simulink model "RCcircuit"  (R2019a)
settings: Solver=ode23t  StartTime=0.0  StopTime=2  MaxStep=1e-6  RelTol=1e-10
libraries: powerlib x7
settings Model: Creator=w0x7ce  LastModifiedBy=w0x7ce
settings SolverCC: AlgebraicLoopSolver=LineSearch

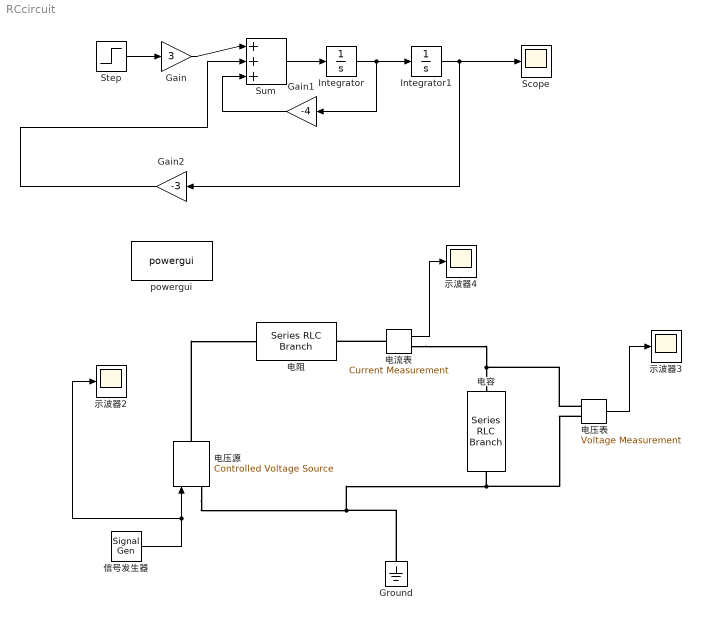
== system RCcircuit ==
  Gain : Gain  Gain=3
  Gain1 : Gain  Gain=-4
  Gain2 : Gain  Gain=-3
  Ground : powerlib/Elements/Ground  LConnTagsString=a
      settings: SourceProductName=Simscape Electrical
  Integrator : Integrator
  Integrator1 : Integrator
  Scope : Scope
  Step : Step  SampleTime=0
  Sum : Sum  Inputs=|+++
  powergui : powerlib/powergui  Priority=1  SimulationMode=Continuous  SampleTime=50e-6  frequency=60  Iterations=50  frequencyindice=0  Pbase=100e6  ErrMax=1e-4  UnitsV=kV  UnitsW=MW  buscounter=0  FunctionMessages=off  echomessages=off  EnableUseOfTLC=off  CurrentSourceSwitches=off  DisableSnubberDevices=off  DisableRonSwitches=off  DisableVfSwitches=off  DisplayEquations=off  AutomaticDiscreteSolvers=off  SolverType=Tustin/Backward Euler (TBE)  Interpol=off  ExternalGateDelay=off  methode=off  Ts=100  x0status=blocks  SPID=on  SwTol=0  HookPort=off  NonlinearTolerance=0  nMaxIteration=15  ContinueOnMaxIteration=off  RestoreLinks=warning  ResistiveCurrentMeasurement=off  Frange=[0:2:500]  Ylog=off  Xlog=on  ShowGrid=off  save=off  variable=ZData  structure=0  ZoomFFT=off  StartTime=0.0  cycles=1  DisplayStyle=1  fundamental=60  FreqAxis=off  MaxFrequency=1000  frequencyindicesteady=1  RmsSteady=1  display=off
      settings: SourceProductName=Simscape Electrical
  信号发生器 : SignalGenerator  WaveForm=square  Amplitude=10  Frequency=2
  电压源 : powerlib/Electrical Sources/Controlled Voltage Source  Initialize=on  Source_Type=AC  Amplitude=0  Phase=0  Frequency=0  Measurements=None
      settings: SourceProductName=Simscape Electrical
  电压表 : powerlib/Measurements/Voltage Measurement  PhasorSimulation=off  OutputType=Complex  PSBequivalent=0
      settings: SourceProductName=Simscape Electrical
  电容 : powerlib/Elements/Series RLC Branch  LConnTagsString=__new0  RConnTagsString=__new0  BranchType=C  Resistance=1  Inductance=1e-3  SetiL0=off  InitialCurrent=0  Capacitance=1e-6  Setx0=off  InitialVoltage=0  Measurements=None
      settings: SourceProductName=Simscape Electrical
  电流表 : powerlib/Measurements/Current Measurement  PhasorSimulation=off  OutputType=Complex  PSBequivalent=0
      settings: SourceProductName=Simscape Electrical
  电阻 : powerlib/Elements/Series RLC Branch  LConnTagsString=__new0  RConnTagsString=__new0  BranchType=R  Resistance=1  Inductance=1e-3  SetiL0=off  InitialCurrent=0  Capacitance=1e-6  Setx0=off  InitialVoltage=0  Measurements=None
      settings: SourceProductName=Simscape Electrical
  示波器2 : Scope
  示波器3 : Scope
  示波器4 : Scope
  wires:
  Step/1 -> Gain/1
  Gain/1 -> Sum/1
  Gain1/1 -> Sum/3
  Gain2/1 -> Sum/2
  Integrator/1 -> Gain1/1, Integrator1/1
  Sum/1 -> Integrator/1
  Integrator1/1 -> Scope/1, Gain2/1
  信号发生器/1 -> 示波器2/1, 电压源/1
  电压表/1 -> 示波器3/1
  电流表/1 -> 示波器4/1
  connections:
  电压源/RConn1 -- 电阻/LConn1
  电压源/LConn1 -- Ground/LConn1 -- 电压表/LConn2 -- 电容/RConn1
  电流表/LConn1 -- 电阻/RConn1
  电流表/RConn1 -- 电压表/LConn1 -- 电容/LConn1
